simulink model "client"  (Simulink 7.0)
settings: Solver=ode1  StartTime=0.0  StopTime=inf  FixedStep=0.001  RelTol=1e-3
libraries: quarc_library x3
settings Model: Creator=colinlea  LastModifiedBy=colinlea  SimulationMode=external  ExtModeTrigDuration=10000
settings SolverCC: PositivePriorityOrder=on
settings RTWCC: SystemTargetFile=quarc_windows.tlc  TemplateMakefile=quarc_default_tmf  Description=QuaRC Win32 Target  ProcessScript=quarc_windows_make_rtw_hook
settings STFCustomTargetCC: TargetPreCompLibLocation=C:\DOCUME~1\ALLUSE~1\APPLIC~1\QuaRC\lib\2007b\windows\release  GenFloatMathFcnCalls=ANSI_C  SystemTargetFile=quarc_windows.tlc
settings GRTTargetCC: TargetPreCompLibLocation=C:\DOCUME~1\ALLUSE~1\APPLIC~1\QuaRC\lib\2007b\windows\release  CompOptLevelCompliant=off  MatFileLogging=off  ExtMode=on  ExtModeMexFile=quarc_comm

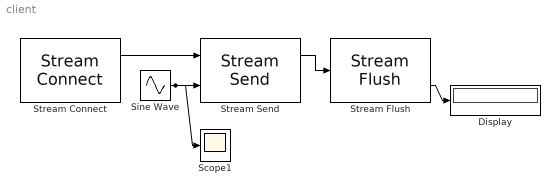
== system client ==
  Display : Display
  Scope1 : Scope
  Sine Wave : Sin  SampleTime=0
  Stream Connect : quarc_library/Communications/Advanced/Stream Connect  uri_source=Internal (dialog parameter)  uri=tcpip://localhost:18000  send_buffer_size=8000  receive_buffer_size=8000  byte_order=little endian (Intel - LSB first)  sample_time=qc_get_step_size  non_blocking=on  active=off
      settings: AttributesFormatString=(%<uri>)
  Stream Flush : quarc_library/Communications/Advanced/Stream Flush
  Stream Send : quarc_library/Communications/Advanced/Stream Send
  wires:
  Stream Connect/1 -> Stream Send/1
  Sine Wave/1 -> Stream Send/2, Scope1/1
  Stream Send/1 -> Stream Flush/1
  Stream Flush/2 -> Display/1
